simulink model "abs"  (R2020b)
settings: Solver=VariableStepAuto  StartTime=0.0  StopTime=10.0  RelTol=1e-3
values from neighbouring files (symbols this model uses):
  ctrl = 1    [dataabs.mat]
  g = 32.18    [dataabs.mat]
  I = 5    [dataabs.mat]
  Kf = 1    [dataabs.mat]
  m = 50    [dataabs.mat]
  mu = [0 0.4 0.8 0.97 1 0.98 0.96 0.94 0.92 0.9 0.88 0.855 ... (21 elements, 1x21)]    [dataabs.mat]
  PBmax = 1500    [dataabs.mat]
  Rr = 1.25    [dataabs.mat]
  slip = [0 0.05 0.1 0.15 0.2 0.25 0.3 0.35 0.4 0.45 0.5 0.55 ... (21 elements, 1x21)]    [dataabs.mat]
  TB = 0.01    [dataabs.mat]
  v0 = 88    [dataabs.mat]
settings Model: Creator=com  LastModifiedBy=com

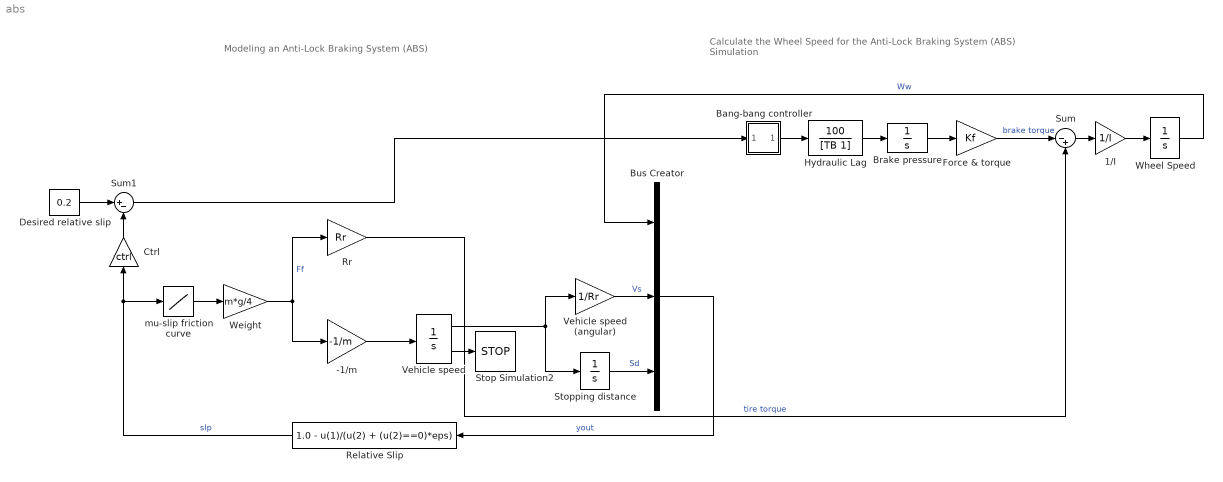
== system abs ==
  note: Modeling an Anti-Lock Braking System (ABS)
  note: Calculate the Wheel Speed for the
      | Anti-Lock Braking System (ABS) Simulation
  -1/m : Gain  Gain=-1/m  SaturateOnIntegerOverflow=on  OutDataTypeStr=Inherit: Same as input  ParamDataTypeStr=Inherit: Same as input
  1/I : Gain  Gain=1/I  SaturateOnIntegerOverflow=on  OutDataTypeStr=Inherit: Same as input  ParamDataTypeStr=Inherit: Same as input
  Bang-bang controller : Subsystem  mask(Sign){}
      mask help: y = sign(x)
      mask Help: Sign Function:\n\t\t\ty = 1 if x > 0\n\t\t\ty = 0 if x = 0\n\t\t\ty = -1 if x < 0
      mask Display: plot(-50,-50,50,50,[-50,50],[0,0],[0,0],[-50,50],[-40,0],[-30,-30],[0,40],[30,30])
  Brake pressure : Integrator  LimitOutput=on  UpperSaturationLimit=PBmax  LowerSaturationLimit=0
  Bus Creator : BusCreator  Inputs=3
  Ctrl : Gain  Gain=ctrl  SaturateOnIntegerOverflow=on  OutDataTypeStr=Inherit: Same as input  ParamDataTypeStr=Inherit: Same as input
  Desired relative slip : Constant  Value=0.2
  Force & torque : Gain  Gain=Kf  SaturateOnIntegerOverflow=on  OutDataTypeStr=Inherit: Same as input  ParamDataTypeStr=Inherit: Same as input
  "Hydraulic Lag " : TransferFcn  Numerator=[100]  Denominator=[TB 1]
  Relative Slip : Fcn  Expr=1.0 - u(1)/(u(2) + (u(2)==0)*eps)
  Rr : Gain  Gain=Rr  SaturateOnIntegerOverflow=on  OutDataTypeStr=Inherit: Same as input  ParamDataTypeStr=Inherit: Same as input
  Stop Simulation2 : Stop
  Stopping distance : Integrator  UpperSaturationLimit=1000  LowerSaturationLimit=0
  Sum : Sum  Inputs=|-+  InputSameDT=on  SaturateOnIntegerOverflow=on  OutDataTypeStr=Inherit: Same as first input
  Sum1 : Sum  Inputs=|+-  InputSameDT=on  SaturateOnIntegerOverflow=on  OutDataTypeStr=Inherit: Same as first input
  Vehicle speed : Integrator  InitialCondition=v0  LimitOutput=on  UpperSaturationLimit=1000  LowerSaturationLimit=0  ShowSaturationPort=on
  Vehicle speed (angular) : Gain  Gain=1/Rr  SaturateOnIntegerOverflow=on  OutDataTypeStr=Inherit: Same as input  ParamDataTypeStr=Inherit: Same as input
  Weight : Gain  Gain=m*g/4  SaturateOnIntegerOverflow=on  OutDataTypeStr=Inherit: Same as input  ParamDataTypeStr=Inherit: Same as input
  Wheel Speed : Integrator  InitialCondition=v0/Rr  LimitOutput=on  UpperSaturationLimit=1000  LowerSaturationLimit=0
  mu-slip friction curve : Lookup_n-D  NumberOfTableDimensions=1  BreakpointsForDimension1=slip  Table=mu  SaturateOnIntegerOverflow=on  InputSameDT=on
  wires:
  Wheel Speed/1 -> Bus Creator/1  "Ww"
  Weight/1 -> -1/m/1, Rr/1  "Ff"
  Desired relative slip/1 -> Sum1/1
  Vehicle speed/2 -> Stop Simulation2/1
  Stopping distance/1 -> Bus Creator/3  "Sd"
  Ctrl/1 -> Sum1/2
  -1/m/1 -> Vehicle speed/1
  Relative Slip/1 -> mu-slip friction curve/1, Ctrl/1  "slp"
  Vehicle speed/1 -> Stopping distance/1, Vehicle speed (angular)/1
  Vehicle speed (angular)/1 -> Bus Creator/2  "Vs"
  Bus Creator/1 -> Relative Slip/1  "yout"
  mu-slip friction curve/1 -> Weight/1
  Bang-bang controller/1(out_1) -> "Hydraulic Lag "/1
  Brake pressure/1 -> Force & torque/1
  Sum/1 -> 1/I/1
  Force & torque/1 -> Sum/1  "brake torque"
  "Hydraulic Lag "/1 -> Brake pressure/1
  1/I/1 -> Wheel Speed/1
  Sum1/1 -> Bang-bang controller/1(in_1)
  Rr/1 -> Sum/2  "tire torque"

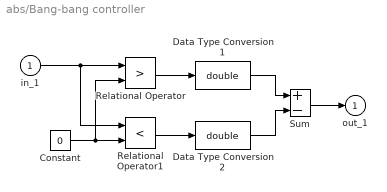
== system abs/Bang-bang controller ==
  in_1 : Inport
  Constant : Constant  Value=0
  Data Type Conversion1 : DataTypeConversion  OutDataTypeStr=double  SaturateOnIntegerOverflow=on  RndMeth=Zero
  Data Type Conversion2 : DataTypeConversion  OutDataTypeStr=double  SaturateOnIntegerOverflow=on  RndMeth=Zero
  Relational Operator : RelationalOperator  Operator=>  OutDataTypeStr=boolean  RndMeth=Nearest  InputSameDT=on
  Relational Operator1 : RelationalOperator  Operator=<  OutDataTypeStr=boolean  RndMeth=Nearest  InputSameDT=on
  Sum : Sum  Inputs=+-  InputSameDT=on  SaturateOnIntegerOverflow=on  OutDataTypeStr=Inherit: Same as first input
  out_1 : Outport  InitialOutput=0  VectorParamsAs1DForOutWhenUnconnected=off
  wires:
  Data Type Conversion2/1 -> Sum/2
  Data Type Conversion1/1 -> Sum/1
  Sum/1 -> out_1/1
  Relational Operator/1 -> Data Type Conversion1/1
  Relational Operator1/1 -> Data Type Conversion2/1
  Constant/1 -> Relational Operator/2, Relational Operator1/2
  in_1/1 -> Relational Operator1/1, Relational Operator/1
